simulink library "Vessel"  (R2023a)
settings: Solver=VariableStepAuto  StartTime=0.0  StopTime=10.0  RelTol=1e-3
undefined symbols (not defined in the file): A_ann_aor, alpha1, alpha2, atrium_ventricle, BSA, control, conversion_factor, DAP, DLVP, DP_close_aor, DP_open_aor, DPP, DRVP, E0, E_max, E_min, E_sa_0, E_sv_0, eta, g, K_vc_aor, K_vo_aor, l, L0, lambda, m1, m2, M_rg_aor, M_st_aor, MAP, MPP, n, P0, p_septum_on_off, p_th_on_off, phi, PVR, Q_max, rho, SAP, SI, sigma, SLVP, SPP, SRVP, SVR, t_delay, Ts, UVV_0, V0, V_0, V_max, V_tot, Y_aorta, Y_control
libraries: $bdroot x100, simulink x39, dspsigops x20, slpidlib x11, eeGeneralControl x2, dspstat3 x1
(part 2 of 4)

== system Vessel/DLVP control1 ==
  DLVP(t) : Inport
  Constant : Constant  Value=DLVP_0
  Constant1 : Constant  Value=onoff
  Data Store Write : DataStoreWrite  DataStoreName=K_LV_Emin  IndexOptions=Index vector (dialog)  Indices=1  OutputSizes=1
  IsZero : simulink/Logic and Bit Operations/Compare To Zero  relop=~=  OutDataTypeStr=boolean
      settings: LibrarySourceBlock=|
      | simulink/Quick Insert/Logic and Bit
      | Operations/IsZero
  IsZero2 : simulink/Logic and Bit Operations/Compare To Zero  relop===  OutDataTypeStr=boolean
      settings: LibrarySourceBlock=|
      | simulink/Quick Insert/Logic and Bit
      | Operations/IsZero
  OR : Logic  Operator=OR  IconShape=distinctive  AllPortsSameDT=off  OutDataTypeStr=boolean
  PID Controller : slpidlib/PID Controller  Controller=PI  Form=Parallel  TimeDomain=Discrete-time  UseExternalTs=off  SampleTime=dt  IntegratorMethod=Forward Euler  FilterMethod=Forward Euler  ControllerParametersSource=internal  P=0.005  I=0.005  UseKiTs=off  D=0.01  N=100  UseFilter=on  TunerSelectOption=Transfer Function Based (PID Tuner App)  InitialConditionSource=internal  InitialConditionForIntegrator=0  InitialConditionForFilter=0  DifferentiatorICPrevScaledInput=0  ExternalReset=either  TrackingMode=off  Kt=1  LimitOutput=on  SatLimitsSource=internal  UpperSaturationLimit=2  LowerSaturationLimit=-0.99  LinearizeAsGain=on  AntiWindupMode=none  Kb=1  LimitIntegrator=off  UpperIntegratorSaturationLimit=inf  LowerIntegratorSaturationLimit=-inf  POutMin=[]  POutMax=[]  IOutMin=[]  IOutMax=[]  DOutMin=[]  DOutMax=[]  NOutMin=[]  NOutMax=[]  SumOutMin=[]  SumOutMax=[]  SaturationOutMin=[]  SaturationOutMax=[]  PParamMin=[]  PParamMax=[]  IParamMin=[]  IParamMax=[]  DParamMin=[]  DParamMax=[]  NParamMin=[]  NParamMax=[]  KbParamMin=[]  KbParamMax=[]  KtParamMin=[]  KtParamMax=[]  KbOutMin=[]  KbOutMax=[]  KtOutMin=[]  KtOutMax=[]  IntegratorOutMin=[]  IntegratorOutMax=[]  FilterOutMin=[]  FilterOutMax=[]  SumI1OutMin=[]  SumI1OutMax=[]  SumI2OutMin=[]  SumI2OutMax=[]  SumI3OutMin=[]  SumI3OutMax=[]  SumI4OutMin=[]  SumI4OutMax=[]  SumDOutMin=[]  SumDOutMax=[]  DifferentiatorOutMin=[]  DifferentiatorOutMax=[]  FilterDiffOutCoefMin=[]  FilterDiffOutCoefMax=[]  ReciprocalOutMin=[]  ReciprocalOutMax=[]  SumDenOutMin=[]  SumDenOutMax=[]  SumNumOutMin=[]  SumNumOutMax=[]  DivideOutMin=[]  DivideOutMax=[]  UdiffTsProdOutMin=[]  UdiffTsProdOutMax=[]  NTsProdOutMin=[]  NTsProdOutMax=[]  UintegralTsProdOutMin=[]  UintegralTsProdOutMax=[]  UngainTsProdOutMin=[]  UngainTsProdOutMax=[]  ClampingZeroOutDataTypeStr=Inherit: Inherit via back propagation  ClampingZeroOutMin=[]  ClampingZeroOutMax=[]  FilterDenConstantOutDataTypeStr=Inherit: Inherit via back propagation  FilterDenConstantOutMin=[]  FilterDenConstantOutMax=[]  PCopyOutDataTypeStr=Inherit: Inherit via back propagation  PCopyOutMin=[]  PCopyOutMax=[]  NCopyOutDataTypeStr=Inherit: Inherit via back propagation  NCopyOutMin=[]  NCopyOutMax=[]  IntegratorContinuousStateAttributes=''  IntegratorStateMustResolveToSignalObject=off  IntegratorRTWStateStorageClass=Auto  FilterContinuousStateAttributes=''  FilterStateMustResolveToSignalObject=off  FilterRTWStateStorageClass=Auto  ParallelPVariant=InternalParameters  IdealPVariant=Disabled  IVariant=InternalParameters  DVariant=Disabled  IntegratorVariant=Discrete  SatVariant=Enabled  AWVariant=Passthrough  PCopyVariant=Disabled  TRVariant=Disabled  FdbkBlocksVariant=Forward  IdealPFdbkVariant=Disabled  SatFdbkVariant=Disabled  DerivativeFilterVariant=Disabled  NVariant=Disabled  NCopyVariant=Disabled_SignalSpec  FilterICVariant=Disabled  IntegratorICVariant=InternalICs  ExternalResetVariant=ExternalReset  TRSumVariant=Passthrough  SumFdbkVariant=Disabled  SumVariant=Sum_PI  TsampFilterVariant=InternalTs  TsampNgainVariant=Passthrough  TsampIntegralVariant=Disabled_SignalSpec  ExternalSaturationOutDataTypeStr=Inherit: Same as second input
  Product : Product
  Subsystem : $bdroot/SLVP control/Subsystem  SystemSampleTime=-1  SSRTWFcnClass=[]  VariantActivationTime=update diagram  Latency=0  AutoFrameSizeCalculation=off
      settings: LibrarySourceBlock=Vessel/SLVP control/Subsystem
  Subtract : Sum  Inputs=+-
  Switch : Switch  Criteria=u2 > Threshold  SaturateOnIntegerOverflow=off  InputSameDT=off
  Switch1 : Switch  Criteria=u2 > Threshold  SaturateOnIntegerOverflow=off  InputSameDT=off
  wires:
  Subtract/1 -> PID Controller/1  "V(t)"
  Constant/1 -> Switch1/3
  [DLVP] -> IsZero2/1, Switch/3
  Switch/1 -> Subtract/2
  IsZero2/1 -> Switch/2
  DLVP(t)/1 -> Switch1/2, IsZero/1, Switch1/1
  Switch1/1 -> Subtract/1, Switch/1
  Product/1 -> Subsystem/2
  IsZero/1 -> OR/2
  Constant1/1 -> OR/1
  OR/1 -> Subsystem/1, Product/1, PID Controller/2
  PID Controller/1 -> Product/2
  Subsystem/1 -> Data Store Write/1

== system Vessel/DRVP control ==
  DRVP(t) : Inport
  Constant : Constant  Value=DRVP_0
  Constant1 : Constant  Value=onoff
  Data Store Write : DataStoreWrite  DataStoreName=K_RV_Emin  IndexOptions=Index vector (dialog)  Indices=1  OutputSizes=1
  IsZero : simulink/Logic and Bit Operations/Compare To Zero  relop=~=  OutDataTypeStr=boolean
      settings: LibrarySourceBlock=|
      | simulink/Quick Insert/Logic and Bit
      | Operations/IsZero
  IsZero2 : simulink/Logic and Bit Operations/Compare To Zero  relop===  OutDataTypeStr=boolean
      settings: LibrarySourceBlock=|
      | simulink/Quick Insert/Logic and Bit
      | Operations/IsZero
  OR : Logic  Operator=OR  IconShape=distinctive  AllPortsSameDT=off  OutDataTypeStr=boolean
  PID Controller : slpidlib/PID Controller  Controller=PI  Form=Parallel  TimeDomain=Discrete-time  UseExternalTs=off  SampleTime=dt  IntegratorMethod=Forward Euler  FilterMethod=Forward Euler  ControllerParametersSource=internal  P=0.005  I=0.005  UseKiTs=off  D=0.01  N=100  UseFilter=on  TunerSelectOption=Transfer Function Based (PID Tuner App)  InitialConditionSource=internal  InitialConditionForIntegrator=0  InitialConditionForFilter=0  DifferentiatorICPrevScaledInput=0  ExternalReset=either  TrackingMode=off  Kt=1  LimitOutput=on  SatLimitsSource=internal  UpperSaturationLimit=2  LowerSaturationLimit=-0.99  LinearizeAsGain=on  AntiWindupMode=none  Kb=1  LimitIntegrator=off  UpperIntegratorSaturationLimit=inf  LowerIntegratorSaturationLimit=-inf  POutMin=[]  POutMax=[]  IOutMin=[]  IOutMax=[]  DOutMin=[]  DOutMax=[]  NOutMin=[]  NOutMax=[]  SumOutMin=[]  SumOutMax=[]  SaturationOutMin=[]  SaturationOutMax=[]  PParamMin=[]  PParamMax=[]  IParamMin=[]  IParamMax=[]  DParamMin=[]  DParamMax=[]  NParamMin=[]  NParamMax=[]  KbParamMin=[]  KbParamMax=[]  KtParamMin=[]  KtParamMax=[]  KbOutMin=[]  KbOutMax=[]  KtOutMin=[]  KtOutMax=[]  IntegratorOutMin=[]  IntegratorOutMax=[]  FilterOutMin=[]  FilterOutMax=[]  SumI1OutMin=[]  SumI1OutMax=[]  SumI2OutMin=[]  SumI2OutMax=[]  SumI3OutMin=[]  SumI3OutMax=[]  SumI4OutMin=[]  SumI4OutMax=[]  SumDOutMin=[]  SumDOutMax=[]  DifferentiatorOutMin=[]  DifferentiatorOutMax=[]  FilterDiffOutCoefMin=[]  FilterDiffOutCoefMax=[]  ReciprocalOutMin=[]  ReciprocalOutMax=[]  SumDenOutMin=[]  SumDenOutMax=[]  SumNumOutMin=[]  SumNumOutMax=[]  DivideOutMin=[]  DivideOutMax=[]  UdiffTsProdOutMin=[]  UdiffTsProdOutMax=[]  NTsProdOutMin=[]  NTsProdOutMax=[]  UintegralTsProdOutMin=[]  UintegralTsProdOutMax=[]  UngainTsProdOutMin=[]  UngainTsProdOutMax=[]  ClampingZeroOutDataTypeStr=Inherit: Inherit via back propagation  ClampingZeroOutMin=[]  ClampingZeroOutMax=[]  FilterDenConstantOutDataTypeStr=Inherit: Inherit via back propagation  FilterDenConstantOutMin=[]  FilterDenConstantOutMax=[]  PCopyOutDataTypeStr=Inherit: Inherit via back propagation  PCopyOutMin=[]  PCopyOutMax=[]  NCopyOutDataTypeStr=Inherit: Inherit via back propagation  NCopyOutMin=[]  NCopyOutMax=[]  IntegratorContinuousStateAttributes=''  IntegratorStateMustResolveToSignalObject=off  IntegratorRTWStateStorageClass=Auto  FilterContinuousStateAttributes=''  FilterStateMustResolveToSignalObject=off  FilterRTWStateStorageClass=Auto  ParallelPVariant=InternalParameters  IdealPVariant=Disabled  IVariant=InternalParameters  DVariant=Disabled  IntegratorVariant=Discrete  SatVariant=Enabled  AWVariant=Passthrough  PCopyVariant=Disabled  TRVariant=Disabled  FdbkBlocksVariant=Forward  IdealPFdbkVariant=Disabled  SatFdbkVariant=Disabled  DerivativeFilterVariant=Disabled  NVariant=Disabled  NCopyVariant=Disabled_SignalSpec  FilterICVariant=Disabled  IntegratorICVariant=InternalICs  ExternalResetVariant=ExternalReset  TRSumVariant=Passthrough  SumFdbkVariant=Disabled  SumVariant=Sum_PI  TsampFilterVariant=InternalTs  TsampNgainVariant=Passthrough  TsampIntegralVariant=Disabled_SignalSpec  ExternalSaturationOutDataTypeStr=Inherit: Same as second input
  Product : Product
  Subsystem : $bdroot/SLVP control/Subsystem  SystemSampleTime=-1  VariantActivationTime=update diagram  Latency=0  AutoFrameSizeCalculation=off
  Subtract : Sum  Inputs=+-
  Switch : Switch  Criteria=u2 > Threshold  SaturateOnIntegerOverflow=off  InputSameDT=off
  Switch1 : Switch  Criteria=u2 > Threshold  SaturateOnIntegerOverflow=off  InputSameDT=off
  wires:
  PID Controller/1 -> Product/2
  OR/1 -> Subsystem/1, PID Controller/2, Product/1
  Constant1/1 -> OR/1
  IsZero/1 -> OR/2
  Product/1 -> Subsystem/2
  Switch1/1 -> Switch/1, Subtract/1
  DRVP(t)/1 -> Switch1/1, IsZero/1, Switch1/2
  IsZero2/1 -> Switch/2
  Switch/1 -> Subtract/2
  [DRVP] -> IsZero2/1, Switch/3
  Constant/1 -> Switch1/3
  Subtract/1 -> PID Controller/1  "V(t)"
  Subsystem/1 -> Data Store Write/1

== system Vessel/Delta to Star conversion ==
  R1 : Inport
  R2 : Inport  Port=2
  R3 : Inport  Port=3
  Add : Sum  Inputs=3
  Divide : Product  Inputs=*/
  Divide1 : Product  Inputs=*/
  Divide2 : Product  Inputs=*/
  Product : Product
  Product1 : Product
  Product2 : Product
  Ra : Outport
  Rb : Outport  Port=2
  Rc : Outport  Port=3
  wires:
  Product1/1 -> Divide/1
  Product2/1 -> Divide1/1
  R1/1 -> Add/2, Product2/1, Product/1
  R2/1 -> Add/3, Product/2, Product1/1
  R3/1 -> Product1/2, Add/1, Product2/2
  Divide/1 -> Ra/1
  Divide1/1 -> Rb/1
  Divide2/1 -> Rc/1
  Add/1 -> Divide1/2, Divide/2, Divide2/2
  Product/1 -> Divide2/1

== system Vessel/Diastolic Pressur ==
  P_in : Inport
  MinMax Running Resettable : simulink/Math Operations/MinMax Running Resettable  Function=min  vinit=300
      settings: AttributesFormatString=%<vinit>
  Pulse Generator1 : DiscretePulseGenerator  PulseType=Time based  TimeSource=Use external signal  Period=100  PulseWidth=1e-3
  Sample and Hold1 : dspsigops/Sample and Hold  trig=Rising edge  initCond=0  latchinput=on
  P_dys : Outport
  wires:
  MinMax Running Resettable/1 -> Sample and Hold1/1
  [t_b] -> Pulse Generator1/1
  P_in/1 -> MinMax Running Resettable/1
  Pulse Generator1/1 -> MinMax Running Resettable/2, Sample and Hold1/Trigger
  Sample and Hold1/1 -> P_dys/1

== system Vessel/Gain ==
  Add : Sum
  Constant : Constant
  Constant1 : Constant  Commented=on  Value=0
  Constant2 : Constant  Commented=on  Value=0
  Constant6 : Constant  Commented=on  Value=control
  Data Store Read : DataStoreRead  Commented=on  DataStoreName=K_svr  IndexOptions=Index vector (dialog)  Indices=1  OutputSizes=1
  Data Store Read1 : DataStoreRead  Commented=on  DataStoreName=K_pvr  IndexOptions=Index vector (dialog)  Indices=1  OutputSizes=1
  Data Store Read2 : DataStoreRead  Commented=on  DataStoreName=K_uvv  IndexOptions=Index vector (dialog)  Indices=1  OutputSizes=1
  Multiport Switch : MultiPortSwitch  Commented=on  Inputs=5  SaturateOnIntegerOverflow=off  InputSameDT=off
  Gain : Outport
  wires:
  Constant2/1 -> Multiport Switch/5
  Constant6/1 -> Multiport Switch/1
  Data Store Read/1 -> Multiport Switch/2
  Add/1 -> Gain/1
  Data Store Read1/1 -> Multiport Switch/3
  Data Store Read2/1 -> Multiport Switch/4
  Constant1/1 -> Multiport Switch/6
  Constant/1 -> Add/1
  Multiport Switch/1 -> Add/2

== system Vessel/Gain UVV ==
  V0 : Inport
  Add : Sum
  Constant : Constant
  Constant1 : Constant  Commented=on  Value=3
  Constant2 : Constant  Commented=on  Value=0
  Constant3 : Constant  Value=0
  Constant4 : Constant  Value=0
  Constant5 : Constant  Value=control
  Constant6 : Constant  Commented=on  Value=control
  Data Store Read : DataStoreRead  DataStoreName=K_svr  IndexOptions=Index vector (dialog)  Indices=1  OutputSizes=1
  Data Store Read1 : DataStoreRead  DataStoreName=K_pvr  IndexOptions=Index vector (dialog)  Indices=1  OutputSizes=1
  Data Store Read2 : DataStoreRead  Commented=on  DataStoreName=K_uvv  IndexOptions=Index vector (dialog)  Indices=1  OutputSizes=1
  Data Store Read3 : DataStoreRead  DataStoreName=K_uvv  IndexOptions=Index vector (dialog)  Indices=1  OutputSizes=1
  Equal : RelationalOperator  Commented=on  Operator===  OutDataTypeStr=boolean  RndMeth=Simplest  InputSameDT=off
  Multiport Switch : MultiPortSwitch  Inputs=5  SaturateOnIntegerOverflow=off  InputSameDT=off
  Product : Product
  Switch : Switch  Commented=on  Criteria=u2 ~= 0  Threshold=3  SaturateOnIntegerOverflow=off  InputSameDT=off
  V0* : Outport
  wires:
  Multiport Switch/1 -> Add/2
  Constant/1 -> Add/1
  Add/1 -> Product/2
  Constant6/1 -> Equal/1
  Constant1/1 -> Equal/2
  Equal/1 -> Switch/2
  Data Store Read2/1 -> Switch/1
  V0/1 -> Product/1
  Product/1 -> V0*/1
  Constant2/1 -> Switch/3
  Constant5/1 -> Multiport Switch/1
  Data Store Read1/1 -> Multiport Switch/3
  Constant4/1 -> Multiport Switch/5
  Data Store Read3/1 -> Multiport Switch/4
  Data Store Read/1 -> Multiport Switch/2
  Constant3/1 -> Multiport Switch/6

== system Vessel/Gain_E_max ==
  E_max : Inport
  Add : Sum
  Constant : Constant
  Constant1 : Constant  Value=0
  Constant2 : Constant  Value=0
  Constant6 : Constant  Value=control
  Data Store Read : DataStoreRead  DataStoreName=K_RA_Emax  IndexOptions=Index vector (dialog)  Indices=1  OutputSizes=1
  Data Store Read1 : DataStoreRead  DataStoreName=K_RV_Emax  IndexOptions=Index vector (dialog)  Indices=1  OutputSizes=1
  Data Store Read2 : DataStoreRead  DataStoreName=K_LA_Emax  IndexOptions=Index vector (dialog)  Indices=1  OutputSizes=1
  Data Store Read3 : DataStoreRead  DataStoreName=K_LV_Emax  IndexOptions=Index vector (dialog)  Indices=1  OutputSizes=1
  Multiport Switch : MultiPortSwitch  Inputs=6  SaturateOnIntegerOverflow=off  InputSameDT=off
  Product : Product
  E_max* : Outport
  wires:
  Multiport Switch/1 -> Add/2
  Constant/1 -> Add/1
  Constant1/1 -> Multiport Switch/7
  Data Store Read2/1 -> Multiport Switch/4
  Data Store Read1/1 -> Multiport Switch/3
  Add/1 -> Product/2
  Data Store Read/1 -> Multiport Switch/2
  Constant6/1 -> Multiport Switch/1
  Data Store Read3/1 -> Multiport Switch/5
  Constant2/1 -> Multiport Switch/6
  Product/1 -> E_max*/1
  E_max/1 -> Product/1

== system Vessel/Gain_E_min ==
  E_min : Inport
  Add : Sum
  Constant : Constant
  Constant1 : Constant  Value=0
  Constant2 : Constant  Value=0
  Constant6 : Constant  Value=control
  Data Store Read : DataStoreRead  DataStoreName=K_RA_Emin  IndexOptions=Index vector (dialog)  Indices=1  OutputSizes=1
  Data Store Read1 : DataStoreRead  DataStoreName=K_RV_Emin  IndexOptions=Index vector (dialog)  Indices=1  OutputSizes=1
  Data Store Read2 : DataStoreRead  DataStoreName=K_LA_Emin  IndexOptions=Index vector (dialog)  Indices=1  OutputSizes=1
  Data Store Read3 : DataStoreRead  DataStoreName=K_LV_Emin  IndexOptions=Index vector (dialog)  Indices=1  OutputSizes=1
  Multiport Switch : MultiPortSwitch  Inputs=6  SaturateOnIntegerOverflow=off  InputSameDT=off
  Product : Product
  E_min* : Outport
  wires:
  E_min/1 -> Product/1
  Product/1 -> E_min*/1
  Constant2/1 -> Multiport Switch/6
  Data Store Read3/1 -> Multiport Switch/5
  Constant6/1 -> Multiport Switch/1
  Data Store Read/1 -> Multiport Switch/2
  Add/1 -> Product/2
  Data Store Read1/1 -> Multiport Switch/3
  Data Store Read2/1 -> Multiport Switch/4
  Constant1/1 -> Multiport Switch/7
  Constant/1 -> Add/1
  Multiport Switch/1 -> Add/2

== system Vessel/Gain_Y ==
  Y : Inport
  Add : Sum
  Constant : Constant
  Constant1 : Constant  Value=0
  Constant2 : Constant  Value=0
  Constant6 : Constant  Value=Y_control
  Data Store Read : DataStoreRead  DataStoreName=K_Y_aorta  IndexOptions=Index vector (dialog)  Indices=1  OutputSizes=1
  Data Store Read1 : DataStoreRead  DataStoreName=K_Y_systemic_veins  IndexOptions=Index vector (dialog)  Indices=1  OutputSizes=1
  Data Store Read2 : DataStoreRead  DataStoreName=K_Y_pulmonary_arteries  IndexOptions=Index vector (dialog)  Indices=1  OutputSizes=1
  Data Store Read3 : DataStoreRead  DataStoreName=K_Y_pulmonary_veins  IndexOptions=Index vector (dialog)  Indices=1  OutputSizes=1
  Multiport Switch : MultiPortSwitch  Inputs=6  SaturateOnIntegerOverflow=off  InputSameDT=off
  Product : Product
  Y* : Outport
  wires:
  Y/1 -> Product/1
  Product/1 -> Y*/1
  Constant2/1 -> Multiport Switch/6
  Data Store Read3/1 -> Multiport Switch/5
  Constant6/1 -> Multiport Switch/1
  Data Store Read/1 -> Multiport Switch/2
  Add/1 -> Product/2
  Data Store Read1/1 -> Multiport Switch/3
  Data Store Read2/1 -> Multiport Switch/4
  Constant1/1 -> Multiport Switch/7
  Constant/1 -> Add/1
  Multiport Switch/1 -> Add/2

== system Vessel/Heart Chamber1 ==
  Q_Input : Inport
  Q_Output : Inport  Port=2
  P_other : Inport  Port=3
  Constant : Constant  Value=p_septum_on_off
  Constant10 : Constant  Value=R_wall
  Constant11 : Constant  Value=v_o
  Constant13 : Constant  Value=V_0
  Delay : Delay  DelayLength=1
  Delay1 : Delay  DelayLength=1  InitialCondition=0
  Integrator : Integrator  InitialConditionSource=external  LimitOutput=on  UpperSaturationLimit=V_max  LowerSaturationLimit=0
  Pericardial pressure : Subsystem
  Product1 : Product  Inputs=3
  Product2 : Product
  Sum1 : Sum  Inputs=+-
  Sum2 : Sum  Inputs=+++
  Sum3 : Sum  Inputs=+-
  Switch : Switch  Criteria=u2 > Threshold  SaturateOnIntegerOverflow=off  InputSameDT=off
  Time varying elastance1 : $bdroot/Time varying elastance1  SystemSampleTime=-1  VariantActivationTime=update diagram  Latency=0  AutoFrameSizeCalculation=off
  Transeptal pressure : $bdroot/Transeptal pressure  SystemSampleTime=-1  VariantActivationTime=update diagram  Latency=0  AutoFrameSizeCalculation=off
  V_ed_new : $bdroot/V_ed_new  SystemSampleTime=-1  VariantActivationTime=update diagram  Latency=0  AutoFrameSizeCalculation=off
  P_Output : Outport
  V : Outport  Port=2
  wires:
  Product2/1 -> Switch/3
  Sum3/1 -> Transeptal pressure/1, Product2/1  "V-V_0"
  Constant13/1 -> Sum3/2
  Integrator/1 -> V_ed_new/1, Time varying elastance1/2, V/1, Sum3/1  "V"
  Constant11/1 -> Integrator/2
  Constant10/1 -> Product1/3
  Sum2/1 -> Delay1/1  "P_chamber"
  Q_Input/1 -> Sum1/1
  Sum1/1 -> Delay/1, Integrator/1  "V'"
  Pericardial pressure/1(P_pc) -> Sum2/3  "P_pc"
  V_ed_new/1 -> Time varying elastance1/1
  Transeptal pressure/1 -> Switch/1
  Constant/1 -> Switch/2
  Switch/1 -> Product1/1, Sum2/1
  P_other/1 -> Transeptal pressure/3
  Delay/1 -> Product1/2
  [V_pc] -> Pericardial pressure/1(Vpc)
  Time varying elastance1/1 -> Product2/2, Transeptal pressure/2
  Product1/1 -> Sum2/2
  Q_Output/1 -> Sum1/2, Time varying elastance1/3
  Delay1/1 -> P_Output/1

== system Vessel/Inductance ==
  r(t) : Inport
  Gain1 : Gain  Gain=rho*l/pi/n/g/conversion_factor
  Math Function : Math  Operator=reciprocal
  Power1 : Math  Operator=square
  L(t) : Outport
  wires:
  Math Function/1 -> Gain1/1
  r(t)/1 -> Power1/1
  Power1/1 -> Math Function/1
  Gain1/1 -> L(t)/1  "L(t)"

== system Vessel/Intrathoracic Pressure ==
  Add : Sum  Inputs=-+
  Add1 : Sum
  Breathing cycle : Subsystem
  Constant : Constant  Value=t_exp
  Constant1 : Constant
  Constant2 : Constant  Value=p_itb
  Constant4 : Constant  Value=t_exp
  Exp : Math
  Exp1 : Math
  Subtract : Sum  Inputs=+-
  Subtract1 : Sum  Inputs=+-
  Switch : Switch  SaturateOnIntegerOverflow=off  InputSameDT=off
  To Workspace4 : ToWorkspace  VariableName=P_Ao1  SampleTime=-1
  amplitude : Gain  Gain=p_ita
  amplitude1 : Gain  Gain=p_ita
  expiration : Gain  Gain=-1/tau_exp
  inspiration : Gain  Gain=-1/tau_insp
  P_ith : Outport
  tag scope: P_ith=global
  wires:
  Switch/1 -> Add1/1
  amplitude1/1 -> Switch/3
  Constant2/1 -> Add1/2
  Add/1 -> amplitude1/1
  Exp/1 -> amplitude/1
  Constant/1 -> Subtract/2
  Subtract/1 -> Switch/2
  Exp1/1 -> Add/1
  expiration/1 -> Exp1/1
  inspiration/1 -> Exp/1
  [t_breathing] -> Subtract/1
  Constant1/1 -> Add/2
  Subtract1/1 -> inspiration/1
  Constant4/1 -> Subtract1/2
  amplitude/1 -> Switch/1
  [t_breathing] -> expiration/1
  [t_breathing] -> Subtract1/1
  Add1/1 -> To Workspace4/1, [P_ith], P_ith/1

== system Vessel/MAP ==
  P_ao : Inport
  Data Store Read1 : DataStoreRead  DataStoreName=T  IndexOptions=Index vector (dialog)  Indices=1  OutputSizes=1
  Divide : Product  Inputs=/*
  Integrator : Integrator  ExternalReset=falling
  Pulse Generator : DiscretePulseGenerator  PulseType=Time based  TimeSource=Use external signal  Period=100  PulseWidth=1e-3
  Sample and Hold : dspsigops/Sample and Hold  trig=Rising edge  initCond=0  latchinput=off
  MAP : Outport
  wires:
  P_ao/1 -> Integrator/1
  Data Store Read1/1 -> Divide/1
  Divide/1 -> MAP/1
  [t_b] -> Pulse Generator/1
  Pulse Generator/1 -> Sample and Hold/Trigger, Integrator/2
  Integrator/1 -> Sample and Hold/1
  Sample and Hold/1 -> Divide/2

== system Vessel/MAP control ==
  MAP(t) : Inport
  Constant : Constant  Value=MAP_0
  Constant1 : Constant  Value=onoff
  Data Store Write : DataStoreWrite  DataStoreName=K_LV_Emax  IndexOptions=Index vector (dialog)  Indices=1  OutputSizes=1
  IsZero : simulink/Logic and Bit Operations/Compare To Zero  relop=~=  OutDataTypeStr=boolean
      settings: LibrarySourceBlock=|
      | simulink/Quick Insert/Logic and Bit
      | Operations/IsZero
  IsZero2 : simulink/Logic and Bit Operations/Compare To Zero  relop===  OutDataTypeStr=boolean
      settings: LibrarySourceBlock=|
      | simulink/Quick Insert/Logic and Bit
      | Operations/IsZero
  OR : Logic  Operator=OR  IconShape=distinctive  AllPortsSameDT=off  OutDataTypeStr=boolean
  PID Controller : slpidlib/PID Controller  Controller=PI  Form=Parallel  TimeDomain=Discrete-time  UseExternalTs=off  SampleTime=dt  IntegratorMethod=Forward Euler  FilterMethod=Forward Euler  ControllerParametersSource=internal  P=0.01  I=0.01  UseKiTs=off  D=0.01  N=100  UseFilter=on  TunerSelectOption=Transfer Function Based (PID Tuner App)  InitialConditionSource=internal  InitialConditionForIntegrator=0  InitialConditionForFilter=0  DifferentiatorICPrevScaledInput=0  ExternalReset=either  TrackingMode=off  Kt=1  LimitOutput=on  SatLimitsSource=internal  UpperSaturationLimit=2  LowerSaturationLimit=-0.99  LinearizeAsGain=on  AntiWindupMode=none  Kb=1  LimitIntegrator=off  UpperIntegratorSaturationLimit=inf  LowerIntegratorSaturationLimit=-inf  POutMin=[]  POutMax=[]  IOutMin=[]  IOutMax=[]  DOutMin=[]  DOutMax=[]  NOutMin=[]  NOutMax=[]  SumOutMin=[]  SumOutMax=[]  SaturationOutMin=[]  SaturationOutMax=[]  PParamMin=[]  PParamMax=[]  IParamMin=[]  IParamMax=[]  DParamMin=[]  DParamMax=[]  NParamMin=[]  NParamMax=[]  KbParamMin=[]  KbParamMax=[]  KtParamMin=[]  KtParamMax=[]  KbOutMin=[]  KbOutMax=[]  KtOutMin=[]  KtOutMax=[]  IntegratorOutMin=[]  IntegratorOutMax=[]  FilterOutMin=[]  FilterOutMax=[]  SumI1OutMin=[]  SumI1OutMax=[]  SumI2OutMin=[]  SumI2OutMax=[]  SumI3OutMin=[]  SumI3OutMax=[]  SumI4OutMin=[]  SumI4OutMax=[]  SumDOutMin=[]  SumDOutMax=[]  DifferentiatorOutMin=[]  DifferentiatorOutMax=[]  FilterDiffOutCoefMin=[]  FilterDiffOutCoefMax=[]  ReciprocalOutMin=[]  ReciprocalOutMax=[]  SumDenOutMin=[]  SumDenOutMax=[]  SumNumOutMin=[]  SumNumOutMax=[]  DivideOutMin=[]  DivideOutMax=[]  UdiffTsProdOutMin=[]  UdiffTsProdOutMax=[]  NTsProdOutMin=[]  NTsProdOutMax=[]  UintegralTsProdOutMin=[]  UintegralTsProdOutMax=[]  UngainTsProdOutMin=[]  UngainTsProdOutMax=[]  ClampingZeroOutDataTypeStr=Inherit: Inherit via back propagation  ClampingZeroOutMin=[]  ClampingZeroOutMax=[]  FilterDenConstantOutDataTypeStr=Inherit: Inherit via back propagation  FilterDenConstantOutMin=[]  FilterDenConstantOutMax=[]  PCopyOutDataTypeStr=Inherit: Inherit via back propagation  PCopyOutMin=[]  PCopyOutMax=[]  NCopyOutDataTypeStr=Inherit: Inherit via back propagation  NCopyOutMin=[]  NCopyOutMax=[]  IntegratorContinuousStateAttributes=''  IntegratorStateMustResolveToSignalObject=off  IntegratorRTWStateStorageClass=Auto  FilterContinuousStateAttributes=''  FilterStateMustResolveToSignalObject=off  FilterRTWStateStorageClass=Auto  ParallelPVariant=InternalParameters  IdealPVariant=Disabled  IVariant=InternalParameters  DVariant=Disabled  IntegratorVariant=Discrete  SatVariant=Enabled  AWVariant=Passthrough  PCopyVariant=Disabled  TRVariant=Disabled  FdbkBlocksVariant=Forward  IdealPFdbkVariant=Disabled  SatFdbkVariant=Disabled  DerivativeFilterVariant=Disabled  NVariant=Disabled  NCopyVariant=Disabled_SignalSpec  FilterICVariant=Disabled  IntegratorICVariant=InternalICs  ExternalResetVariant=ExternalReset  TRSumVariant=Passthrough  SumFdbkVariant=Disabled  SumVariant=Sum_PI  TsampFilterVariant=InternalTs  TsampNgainVariant=Passthrough  TsampIntegralVariant=Disabled_SignalSpec  ExternalSaturationOutDataTypeStr=Inherit: Same as second input
  Product : Product
  Subsystem : $bdroot/SLVP control/Subsystem  SystemSampleTime=-1  VariantActivationTime=update diagram  Latency=0  AutoFrameSizeCalculation=off
  Subtract : Sum  Inputs=+-
  Switch : Switch  Criteria=u2 > Threshold  SaturateOnIntegerOverflow=off  InputSameDT=off
  Switch1 : Switch  Criteria=u2 > Threshold  SaturateOnIntegerOverflow=off  InputSameDT=off
  wires:
  Subtract/1 -> PID Controller/1  "V(t)"
  Constant/1 -> Switch1/3
  [MAP] -> IsZero2/1, Switch/3
  Switch/1 -> Subtract/2
  IsZero2/1 -> Switch/2
  MAP(t)/1 -> Switch1/2, IsZero/1, Switch1/1
  Switch1/1 -> Subtract/1, Switch/1
  Product/1 -> Subsystem/2
  IsZero/1 -> OR/2
  Constant1/1 -> OR/1
  OR/1 -> Subsystem/1, Product/1, PID Controller/2
  PID Controller/1 -> Product/2
  Subsystem/1 -> Data Store Write/1

== system Vessel/MPP control ==
  MPP(t) : Inport
  Constant : Constant  Value=MPP_0
  Constant1 : Constant  Value=onoff
  Data Store Write : DataStoreWrite  DataStoreName=K_RV_Emax  IndexOptions=Index vector (dialog)  Indices=1  OutputSizes=1
  IsZero : simulink/Logic and Bit Operations/Compare To Zero  relop=~=  OutDataTypeStr=boolean
      settings: LibrarySourceBlock=|
      | simulink/Quick Insert/Logic and Bit
      | Operations/IsZero
  IsZero2 : simulink/Logic and Bit Operations/Compare To Zero  relop===  OutDataTypeStr=boolean
      settings: LibrarySourceBlock=|
      | simulink/Quick Insert/Logic and Bit
      | Operations/IsZero
  OR : Logic  Operator=OR  IconShape=distinctive  AllPortsSameDT=off  OutDataTypeStr=boolean
  PID Controller : slpidlib/PID Controller  Controller=PI  Form=Parallel  TimeDomain=Discrete-time  UseExternalTs=off  SampleTime=dt  IntegratorMethod=Forward Euler  FilterMethod=Forward Euler  ControllerParametersSource=internal  P=0.005  I=0.005  UseKiTs=off  D=0.01  N=100  UseFilter=on  TunerSelectOption=Transfer Function Based (PID Tuner App)  InitialConditionSource=internal  InitialConditionForIntegrator=0  InitialConditionForFilter=0  DifferentiatorICPrevScaledInput=0  ExternalReset=either  TrackingMode=off  Kt=1  LimitOutput=on  SatLimitsSource=internal  UpperSaturationLimit=2  LowerSaturationLimit=-0.99  LinearizeAsGain=on  AntiWindupMode=none  Kb=1  LimitIntegrator=off  UpperIntegratorSaturationLimit=inf  LowerIntegratorSaturationLimit=-inf  POutMin=[]  POutMax=[]  IOutMin=[]  IOutMax=[]  DOutMin=[]  DOutMax=[]  NOutMin=[]  NOutMax=[]  SumOutMin=[]  SumOutMax=[]  SaturationOutMin=[]  SaturationOutMax=[]  PParamMin=[]  PParamMax=[]  IParamMin=[]  IParamMax=[]  DParamMin=[]  DParamMax=[]  NParamMin=[]  NParamMax=[]  KbParamMin=[]  KbParamMax=[]  KtParamMin=[]  KtParamMax=[]  KbOutMin=[]  KbOutMax=[]  KtOutMin=[]  KtOutMax=[]  IntegratorOutMin=[]  IntegratorOutMax=[]  FilterOutMin=[]  FilterOutMax=[]  SumI1OutMin=[]  SumI1OutMax=[]  SumI2OutMin=[]  SumI2OutMax=[]  SumI3OutMin=[]  SumI3OutMax=[]  SumI4OutMin=[]  SumI4OutMax=[]  SumDOutMin=[]  SumDOutMax=[]  DifferentiatorOutMin=[]  DifferentiatorOutMax=[]  FilterDiffOutCoefMin=[]  FilterDiffOutCoefMax=[]  ReciprocalOutMin=[]  ReciprocalOutMax=[]  SumDenOutMin=[]  SumDenOutMax=[]  SumNumOutMin=[]  SumNumOutMax=[]  DivideOutMin=[]  DivideOutMax=[]  UdiffTsProdOutMin=[]  UdiffTsProdOutMax=[]  NTsProdOutMin=[]  NTsProdOutMax=[]  UintegralTsProdOutMin=[]  UintegralTsProdOutMax=[]  UngainTsProdOutMin=[]  UngainTsProdOutMax=[]  ClampingZeroOutDataTypeStr=Inherit: Inherit via back propagation  ClampingZeroOutMin=[]  ClampingZeroOutMax=[]  FilterDenConstantOutDataTypeStr=Inherit: Inherit via back propagation  FilterDenConstantOutMin=[]  FilterDenConstantOutMax=[]  PCopyOutDataTypeStr=Inherit: Inherit via back propagation  PCopyOutMin=[]  PCopyOutMax=[]  NCopyOutDataTypeStr=Inherit: Inherit via back propagation  NCopyOutMin=[]  NCopyOutMax=[]  IntegratorContinuousStateAttributes=''  IntegratorStateMustResolveToSignalObject=off  IntegratorRTWStateStorageClass=Auto  FilterContinuousStateAttributes=''  FilterStateMustResolveToSignalObject=off  FilterRTWStateStorageClass=Auto  ParallelPVariant=InternalParameters  IdealPVariant=Disabled  IVariant=InternalParameters  DVariant=Disabled  IntegratorVariant=Discrete  SatVariant=Enabled  AWVariant=Passthrough  PCopyVariant=Disabled  TRVariant=Disabled  FdbkBlocksVariant=Forward  IdealPFdbkVariant=Disabled  SatFdbkVariant=Disabled  DerivativeFilterVariant=Disabled  NVariant=Disabled  NCopyVariant=Disabled_SignalSpec  FilterICVariant=Disabled  IntegratorICVariant=InternalICs  ExternalResetVariant=ExternalReset  TRSumVariant=Passthrough  SumFdbkVariant=Disabled  SumVariant=Sum_PI  TsampFilterVariant=InternalTs  TsampNgainVariant=Passthrough  TsampIntegralVariant=Disabled_SignalSpec  ExternalSaturationOutDataTypeStr=Inherit: Same as second input
  Product : Product
  Subsystem : $bdroot/SLVP control/Subsystem  SystemSampleTime=-1  VariantActivationTime=update diagram  Latency=0  AutoFrameSizeCalculation=off
  Subtract : Sum  Inputs=+-
  Switch : Switch  Criteria=u2 > Threshold  SaturateOnIntegerOverflow=off  InputSameDT=off
  Switch1 : Switch  Criteria=u2 > Threshold  SaturateOnIntegerOverflow=off  InputSameDT=off
  wires:
  PID Controller/1 -> Product/2
  OR/1 -> Subsystem/1, PID Controller/2, Product/1
  Constant1/1 -> OR/1
  IsZero/1 -> OR/2
  Product/1 -> Subsystem/2
  Switch1/1 -> Switch/1, Subtract/1
  MPP(t)/1 -> Switch1/1, IsZero/1, Switch1/2
  IsZero2/1 -> Switch/2
  Switch/1 -> Subtract/2
  [MPP] -> IsZero2/1, Switch/3
  Constant/1 -> Switch1/3
  Subtract/1 -> PID Controller/1  "V(t)"
  Subsystem/1 -> Data Store Write/1

== system Vessel/Omega ==
  V-V0 : Inport  Unit=mL
  L(t) : Inport  Port=2  Unit=mmHg*s^2/mL
  Constant : Constant  Value=E0
  Constant1 : Constant  Value=L0
  Constant9 : Constant  Value=lambda
  Product : Product
  Product9 : Product
  Sqrt : Sqrt
  Subsystem : Subsystem
  Switch1 : Switch  Criteria=u2 ~= 0  SaturateOnIntegerOverflow=off  InputSameDT=off
  Switch2 : Switch  Criteria=u2 > Threshold  SaturateOnIntegerOverflow=off  InputSameDT=off
  Ω : Outport
  wires:
  Product/1 -> Ω/1
  Constant9/1 -> Product/2
  V-V0/1 -> Switch1/2, Subsystem/1(V-V0)
  L(t)/1 -> Switch2/2, Switch2/1
  Switch1/1 -> Product9/1  "E(t)"
  Sqrt/1 -> Product/1
  Product9/1 -> Sqrt/1
  Subsystem/1(E(t)) -> Switch1/1  "E(t)"
  Constant/1 -> Switch1/3
  Switch2/1 -> Product9/2  "L(t)"
  Constant1/1 -> Switch2/3

== system Vessel/PVR Control ==
  PVR(t) : Inport
  Constant : Constant  Value=PVR_0
  Constant1 : Constant  Value=0
  Data Store Write : DataStoreWrite  DataStoreName=K_pvr  IndexOptions=Index vector (dialog)  Indices=1  OutputSizes=1
  IsZero1 : simulink/Logic and Bit Operations/Compare To Zero  relop=~=  OutDataTypeStr=boolean
      settings: LibrarySourceBlock=|
      | simulink/Quick Insert/Logic and Bit
      | Operations/IsZero
  K_pvr : Constant  Value=0
  MATLAB Function : MATLAB Function  TreatAsAtomicUnit=on
  OR : Logic  Operator=OR  IconShape=distinctive  AllPortsSameDT=off  OutDataTypeStr=boolean
  PID Controller : slpidlib/PID Controller  Controller=PI  Form=Parallel  TimeDomain=Continuous-time  UseExternalTs=off  SampleTime=-1  IntegratorMethod=Forward Euler  FilterMethod=Forward Euler  ControllerParametersSource=internal  P=0.3  I=0.3  UseKiTs=off  D=0.01  N=100  UseFilter=on  TunerSelectOption=Transfer Function Based (PID Tuner App)  InitialConditionSource=internal  InitialConditionForIntegrator=0  InitialConditionForFilter=0  DifferentiatorICPrevScaledInput=0  ExternalReset=either  TrackingMode=off  Kt=1  LimitOutput=off  SatLimitsSource=internal  UpperSaturationLimit=inf  LowerSaturationLimit=-inf  LinearizeAsGain=on  AntiWindupMode=none  Kb=1  LimitIntegrator=off  UpperIntegratorSaturationLimit=inf  LowerIntegratorSaturationLimit=-inf  POutMin=[]  POutMax=[]  IOutMin=[]  IOutMax=[]  DOutMin=[]  DOutMax=[]  NOutMin=[]  NOutMax=[]  SumOutMin=[]  SumOutMax=[]  SaturationOutMin=[]  SaturationOutMax=[]  PParamMin=[]  PParamMax=[]  IParamMin=[]  IParamMax=[]  DParamMin=[]  DParamMax=[]  NParamMin=[]  NParamMax=[]  KbParamMin=[]  KbParamMax=[]  KtParamMin=[]  KtParamMax=[]  KbOutMin=[]  KbOutMax=[]  KtOutMin=[]  KtOutMax=[]  IntegratorOutMin=[]  IntegratorOutMax=[]  FilterOutMin=[]  FilterOutMax=[]  SumI1OutMin=[]  SumI1OutMax=[]  SumI2OutMin=[]  SumI2OutMax=[]  SumI3OutMin=[]  SumI3OutMax=[]  SumI4OutMin=[]  SumI4OutMax=[]  SumDOutMin=[]  SumDOutMax=[]  DifferentiatorOutMin=[]  DifferentiatorOutMax=[]  FilterDiffOutCoefMin=[]  FilterDiffOutCoefMax=[]  ReciprocalOutMin=[]  ReciprocalOutMax=[]  SumDenOutMin=[]  SumDenOutMax=[]  SumNumOutMin=[]  SumNumOutMax=[]  DivideOutMin=[]  DivideOutMax=[]  UdiffTsProdOutMin=[]  UdiffTsProdOutMax=[]  NTsProdOutMin=[]  NTsProdOutMax=[]  UintegralTsProdOutMin=[]  UintegralTsProdOutMax=[]  UngainTsProdOutMin=[]  UngainTsProdOutMax=[]  ClampingZeroOutDataTypeStr=Inherit: Inherit via back propagation  ClampingZeroOutMin=[]  ClampingZeroOutMax=[]  FilterDenConstantOutDataTypeStr=Inherit: Inherit via back propagation  FilterDenConstantOutMin=[]  FilterDenConstantOutMax=[]  PCopyOutDataTypeStr=Inherit: Inherit via back propagation  PCopyOutMin=[]  PCopyOutMax=[]  NCopyOutDataTypeStr=Inherit: Inherit via back propagation  NCopyOutMin=[]  NCopyOutMax=[]  IntegratorContinuousStateAttributes=''  IntegratorStateMustResolveToSignalObject=off  IntegratorRTWStateStorageClass=Auto  FilterContinuousStateAttributes=''  FilterStateMustResolveToSignalObject=off  FilterRTWStateStorageClass=Auto  ParallelPVariant=InternalParameters  IdealPVariant=Disabled  IVariant=InternalParameters  DVariant=Disabled  IntegratorVariant=Continuous  SatVariant=Disabled  AWVariant=Passthrough  PCopyVariant=Disabled  TRVariant=Disabled  FdbkBlocksVariant=Forward  IdealPFdbkVariant=Disabled  SatFdbkVariant=Disabled  DerivativeFilterVariant=Disabled  NVariant=Disabled  NCopyVariant=Disabled_SignalSpec  FilterICVariant=Disabled  IntegratorICVariant=InternalICs  ExternalResetVariant=ExternalReset  TRSumVariant=Passthrough  SumFdbkVariant=Disabled  SumVariant=Sum_PI  TsampFilterVariant=InternalTs  TsampNgainVariant=Passthrough  TsampIntegralVariant=Disabled_SignalSpec  ExternalSaturationOutDataTypeStr=Inherit: Same as second input
  Subsystem1 : $bdroot/SVR Control/Subsystem1  SystemSampleTime=-1  VariantActivationTime=update diagram  Latency=0  AutoFrameSizeCalculation=off
  Subsystem2 : $bdroot/SVR Control/Subsystem2  SystemSampleTime=-1  VariantActivationTime=update diagram  Latency=0  AutoFrameSizeCalculation=off
  Subtract : Sum  Inputs=-+
  Switch : Switch  Criteria=u2 > Threshold  SaturateOnIntegerOverflow=off  InputSameDT=off
  Switch1 : Switch  Criteria=u2 > Threshold  SaturateOnIntegerOverflow=off  InputSameDT=off
  Switch2 : Switch  Criteria=u2 > Threshold  SaturateOnIntegerOverflow=off  InputSameDT=off
  Unit Delay2 : UnitDelay  SampleTime=-1  HasFrameUpgradeWarning=on
  wires:
  Switch/1 -> Subtract/2
  Subtract/1 -> PID Controller/1  "V(t)"
  [PVR] -> Subsystem1/1, Switch/3
  Switch1/1 -> Subtract/1, Switch/1
  Subsystem1/1 -> Switch/2
  Constant/1 -> Switch1/3
  Constant1/1 -> OR/1
  PVR(t)/1 -> Switch1/2, IsZero1/1, Switch1/1
  IsZero1/1 -> OR/2
  Switch2/1 -> Data Store Write/1
  K_pvr/1 -> Switch2/3
  OR/1 -> PID Controller/2, MATLAB Function/Trigger, Unit Delay2/1, Subsystem2/2
  PID Controller/1 -> Subsystem2/1
  Unit Delay2/1 -> Switch2/2
  Subsystem2/1 -> MATLAB Function/1(u), Switch2/1

== system Vessel/Radius ==
  V(t) : Inport  Unit=mL
  Gain : Gain  Gain=1/(pi*l*n)
  Gain1 : $bdroot/Gain  SystemSampleTime=-1  VariantActivationTime=update diagram  Latency=0  AutoFrameSizeCalculation=off
  Product : Product
  Sqrt : Sqrt
  r(t) : Outport  Unit=cm
  wires:
  Gain/1 -> Sqrt/1
  Sqrt/1 -> Product/1
  V(t)/1 -> Gain/1
  Gain1/1 -> Product/2
  Product/1 -> r(t)/1

== system Vessel/Resistance ==
  r(t) : Inport
  Gain : Gain  Gain=eta*8*l/(pi*n)*1.1732
  Math Function : Math  Operator=reciprocal
  Power : Math  Operator=square
  Power1 : Math  Operator=square
  R(t) : Outport
  wires:
  r(t)/1 -> Power/1
  Power/1 -> Power1/1
  Power1/1 -> Math Function/1
  Math Function/1 -> Gain/1
  Gain/1 -> R(t)/1  "R(t)"

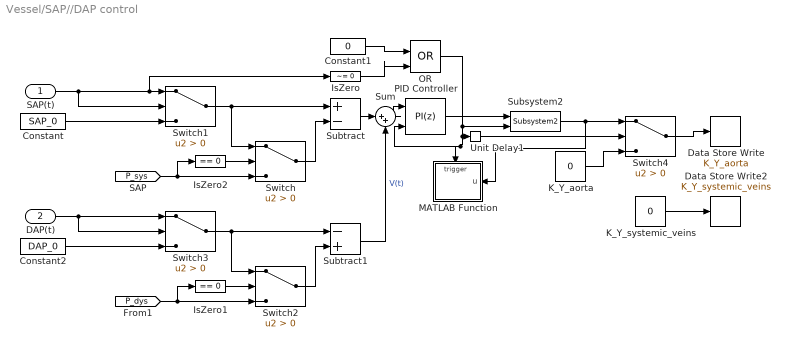
== system Vessel/SAP//DAP control ==
  SAP(t) : Inport
  DAP(t) : Inport  Port=2
  Constant : Constant  Value=SAP_0
  Constant1 : Constant  Value=0
  Constant2 : Constant  Value=DAP_0
  Data Store Write : DataStoreWrite  DataStoreName=K_Y_aorta  IndexOptions=Index vector (dialog)  Indices=1  OutputSizes=1
  Data Store Write2 : DataStoreWrite  DataStoreName=K_Y_systemic_veins  IndexOptions=Index vector (dialog)  Indices=1  OutputSizes=1
  IsZero : simulink/Logic and Bit Operations/Compare To Zero  relop=~=  OutDataTypeStr=boolean
      settings: LibrarySourceBlock=|
      | simulink/Quick Insert/Logic and Bit
      | Operations/IsZero
  IsZero1 : simulink/Logic and Bit Operations/Compare To Zero  relop===  OutDataTypeStr=boolean
      settings: LibrarySourceBlock=|
      | simulink/Quick Insert/Logic and Bit
      | Operations/IsZero
  IsZero2 : simulink/Logic and Bit Operations/Compare To Zero  relop===  OutDataTypeStr=boolean
      settings: LibrarySourceBlock=|
      | simulink/Quick Insert/Logic and Bit
      | Operations/IsZero
  K_Y_aorta : Constant  Value=0
  K_Y_systemic_veins : Constant  Value=0
  MATLAB Function : MATLAB Function  TreatAsAtomicUnit=on
  OR : Logic  Operator=OR  IconShape=distinctive  AllPortsSameDT=off  OutDataTypeStr=boolean
  PID Controller : slpidlib/PID Controller  Controller=PI  Form=Parallel  TimeDomain=Discrete-time  UseExternalTs=off  SampleTime=dt  IntegratorMethod=Forward Euler  FilterMethod=Forward Euler  ControllerParametersSource=internal  P=0.01  I=0.01  UseKiTs=off  D=0.01  N=100  UseFilter=on  TunerSelectOption=Transfer Function Based (PID Tuner App)  InitialConditionSource=internal  InitialConditionForIntegrator=0  InitialConditionForFilter=0  DifferentiatorICPrevScaledInput=0  ExternalReset=either  TrackingMode=off  Kt=1  LimitOutput=on  SatLimitsSource=internal  UpperSaturationLimit=2  LowerSaturationLimit=-0.99  LinearizeAsGain=on  AntiWindupMode=none  Kb=1  LimitIntegrator=off  UpperIntegratorSaturationLimit=inf  LowerIntegratorSaturationLimit=-inf  POutMin=[]  POutMax=[]  IOutMin=[]  IOutMax=[]  DOutMin=[]  DOutMax=[]  NOutMin=[]  NOutMax=[]  SumOutMin=[]  SumOutMax=[]  SaturationOutMin=[]  SaturationOutMax=[]  PParamMin=[]  PParamMax=[]  IParamMin=[]  IParamMax=[]  DParamMin=[]  DParamMax=[]  NParamMin=[]  NParamMax=[]  KbParamMin=[]  KbParamMax=[]  KtParamMin=[]  KtParamMax=[]  KbOutMin=[]  KbOutMax=[]  KtOutMin=[]  KtOutMax=[]  IntegratorOutMin=[]  IntegratorOutMax=[]  FilterOutMin=[]  FilterOutMax=[]  SumI1OutMin=[]  SumI1OutMax=[]  SumI2OutMin=[]  SumI2OutMax=[]  SumI3OutMin=[]  SumI3OutMax=[]  SumI4OutMin=[]  SumI4OutMax=[]  SumDOutMin=[]  SumDOutMax=[]  DifferentiatorOutMin=[]  DifferentiatorOutMax=[]  FilterDiffOutCoefMin=[]  FilterDiffOutCoefMax=[]  ReciprocalOutMin=[]  ReciprocalOutMax=[]  SumDenOutMin=[]  SumDenOutMax=[]  SumNumOutMin=[]  SumNumOutMax=[]  DivideOutMin=[]  DivideOutMax=[]  UdiffTsProdOutMin=[]  UdiffTsProdOutMax=[]  NTsProdOutMin=[]  NTsProdOutMax=[]  UintegralTsProdOutMin=[]  UintegralTsProdOutMax=[]  UngainTsProdOutMin=[]  UngainTsProdOutMax=[]  ClampingZeroOutDataTypeStr=Inherit: Inherit via back propagation  ClampingZeroOutMin=[]  ClampingZeroOutMax=[]  FilterDenConstantOutDataTypeStr=Inherit: Inherit via back propagation  FilterDenConstantOutMin=[]  FilterDenConstantOutMax=[]  PCopyOutDataTypeStr=Inherit: Inherit via back propagation  PCopyOutMin=[]  PCopyOutMax=[]  NCopyOutDataTypeStr=Inherit: Inherit via back propagation  NCopyOutMin=[]  NCopyOutMax=[]  IntegratorContinuousStateAttributes=''  IntegratorStateMustResolveToSignalObject=off  IntegratorRTWStateStorageClass=Auto  FilterContinuousStateAttributes=''  FilterStateMustResolveToSignalObject=off  FilterRTWStateStorageClass=Auto  ParallelPVariant=InternalParameters  IdealPVariant=Disabled  IVariant=InternalParameters  DVariant=Disabled  IntegratorVariant=Discrete  SatVariant=Enabled  AWVariant=Passthrough  PCopyVariant=Disabled  TRVariant=Disabled  FdbkBlocksVariant=Forward  IdealPFdbkVariant=Disabled  SatFdbkVariant=Disabled  DerivativeFilterVariant=Disabled  NVariant=Disabled  NCopyVariant=Disabled_SignalSpec  FilterICVariant=Disabled  IntegratorICVariant=InternalICs  ExternalResetVariant=ExternalReset  TRSumVariant=Passthrough  SumFdbkVariant=Disabled  SumVariant=Sum_PI  TsampFilterVariant=InternalTs  TsampNgainVariant=Passthrough  TsampIntegralVariant=Disabled_SignalSpec  ExternalSaturationOutDataTypeStr=Inherit: Same as second input
  Subsystem2 : $bdroot/SVR Control/Subsystem2  SystemSampleTime=-1  VariantActivationTime=update diagram  Latency=0  AutoFrameSizeCalculation=off
  Subtract : Sum  Inputs=+-
  Subtract1 : Sum  Inputs=-+
  Sum : Sum  Inputs=|++
  Switch{,1..4} (5 alike) : Switch  Criteria=u2 > Threshold  SaturateOnIntegerOverflow=off  InputSameDT=off
  Unit Delay1 : UnitDelay  SampleTime=-1  HasFrameUpgradeWarning=on
  wires:
  Constant/1 -> Switch1/3
  [P_sys] -> IsZero2/1, Switch/3
  Switch/1 -> Subtract/2
  IsZero2/1 -> Switch/2
  SAP(t)/1 -> Switch1/2, IsZero/1, Switch1/1
  Switch1/1 -> Subtract/1, Switch/1
  IsZero/1 -> OR/2
  Constant1/1 -> OR/1
  [P_dys] -> IsZero1/1, Switch2/3
  DAP(t)/1 -> Switch3/1, Switch3/2
  Switch2/1 -> Subtract1/2
  IsZero1/1 -> Switch2/2
  Subtract1/1 -> Sum/2  "V(t)"
  Constant2/1 -> Switch3/3
  Switch3/1 -> Switch2/1, Subtract1/1
  Subtract/1 -> Sum/1
  Sum/1 -> PID Controller/1
  Switch4/1 -> Data Store Write/1
  K_Y_aorta/1 -> Switch4/3
  K_Y_systemic_veins/1 -> Data Store Write2/1
  OR/1 -> Unit Delay1/1, PID Controller/2, MATLAB Function/Trigger, Subsystem2/2
  PID Controller/1 -> Subsystem2/1
  Subsystem2/1 -> Switch4/1, MATLAB Function/1(u)
  Unit Delay1/1 -> Switch4/2

== system Vessel/SLVP control ==
  SLVP(t) : Inport
  Constant : Constant  Value=SLVP_0
  Constant1 : Constant  Value=0
  Data Store Write : DataStoreWrite  DataStoreName=K_LV_Emax  IndexOptions=Index vector (dialog)  Indices=1  OutputSizes=1
  Data Store Write11 : DataStoreWrite  DataStoreName=K_LV_Emin  IndexOptions=Index vector (dialog)  Indices=1  OutputSizes=1
  Data Store Write7 : DataStoreWrite  DataStoreName=K_LA_Emax  IndexOptions=Index vector (dialog)  Indices=1  OutputSizes=1
  Data Store Write8 : DataStoreWrite  DataStoreName=K_LA_Emin  IndexOptions=Index vector (dialog)  Indices=1  OutputSizes=1
  IsZero : simulink/Logic and Bit Operations/Compare To Zero  relop=~=  OutDataTypeStr=boolean
      settings: LibrarySourceBlock=|
      | simulink/Quick Insert/Logic and Bit
      | Operations/IsZero
  IsZero2 : simulink/Logic and Bit Operations/Compare To Zero  relop===  OutDataTypeStr=boolean
      settings: LibrarySourceBlock=|
      | simulink/Quick Insert/Logic and Bit
      | Operations/IsZero
  K_LA_Emax : Constant  Value=0
  K_LA_Emin : Constant  Value=0
  K_LV_Emax : Constant  Value=0
  K_LV_Emin : Constant  Value=0
  MATLAB Function : MATLAB Function  TreatAsAtomicUnit=on
  OR : Logic  Operator=OR  IconShape=distinctive  AllPortsSameDT=off  OutDataTypeStr=boolean
  PID Controller : slpidlib/PID Controller  Controller=PI  Form=Parallel  TimeDomain=Discrete-time  UseExternalTs=off  SampleTime=dt  IntegratorMethod=Forward Euler  FilterMethod=Forward Euler  ControllerParametersSource=internal  P=0.005  I=0.005  UseKiTs=off  D=0.01  N=100  UseFilter=on  TunerSelectOption=Transfer Function Based (PID Tuner App)  InitialConditionSource=internal  InitialConditionForIntegrator=0  InitialConditionForFilter=0  DifferentiatorICPrevScaledInput=0  ExternalReset=either  TrackingMode=off  Kt=1  LimitOutput=on  SatLimitsSource=internal  UpperSaturationLimit=2  LowerSaturationLimit=-0.99  LinearizeAsGain=on  AntiWindupMode=none  Kb=1  LimitIntegrator=off  UpperIntegratorSaturationLimit=inf  LowerIntegratorSaturationLimit=-inf  POutMin=[]  POutMax=[]  IOutMin=[]  IOutMax=[]  DOutMin=[]  DOutMax=[]  NOutMin=[]  NOutMax=[]  SumOutMin=[]  SumOutMax=[]  SaturationOutMin=[]  SaturationOutMax=[]  PParamMin=[]  PParamMax=[]  IParamMin=[]  IParamMax=[]  DParamMin=[]  DParamMax=[]  NParamMin=[]  NParamMax=[]  KbParamMin=[]  KbParamMax=[]  KtParamMin=[]  KtParamMax=[]  KbOutMin=[]  KbOutMax=[]  KtOutMin=[]  KtOutMax=[]  IntegratorOutMin=[]  IntegratorOutMax=[]  FilterOutMin=[]  FilterOutMax=[]  SumI1OutMin=[]  SumI1OutMax=[]  SumI2OutMin=[]  SumI2OutMax=[]  SumI3OutMin=[]  SumI3OutMax=[]  SumI4OutMin=[]  SumI4OutMax=[]  SumDOutMin=[]  SumDOutMax=[]  DifferentiatorOutMin=[]  DifferentiatorOutMax=[]  FilterDiffOutCoefMin=[]  FilterDiffOutCoefMax=[]  ReciprocalOutMin=[]  ReciprocalOutMax=[]  SumDenOutMin=[]  SumDenOutMax=[]  SumNumOutMin=[]  SumNumOutMax=[]  DivideOutMin=[]  DivideOutMax=[]  UdiffTsProdOutMin=[]  UdiffTsProdOutMax=[]  NTsProdOutMin=[]  NTsProdOutMax=[]  UintegralTsProdOutMin=[]  UintegralTsProdOutMax=[]  UngainTsProdOutMin=[]  UngainTsProdOutMax=[]  ClampingZeroOutDataTypeStr=Inherit: Inherit via back propagation  ClampingZeroOutMin=[]  ClampingZeroOutMax=[]  FilterDenConstantOutDataTypeStr=Inherit: Inherit via back propagation  FilterDenConstantOutMin=[]  FilterDenConstantOutMax=[]  PCopyOutDataTypeStr=Inherit: Inherit via back propagation  PCopyOutMin=[]  PCopyOutMax=[]  NCopyOutDataTypeStr=Inherit: Inherit via back propagation  NCopyOutMin=[]  NCopyOutMax=[]  IntegratorContinuousStateAttributes=''  IntegratorStateMustResolveToSignalObject=off  IntegratorRTWStateStorageClass=Auto  FilterContinuousStateAttributes=''  FilterStateMustResolveToSignalObject=off  FilterRTWStateStorageClass=Auto  ParallelPVariant=InternalParameters  IdealPVariant=Disabled  IVariant=InternalParameters  DVariant=Disabled  IntegratorVariant=Discrete  SatVariant=Enabled  AWVariant=Passthrough  PCopyVariant=Disabled  TRVariant=Disabled  FdbkBlocksVariant=Forward  IdealPFdbkVariant=Disabled  SatFdbkVariant=Disabled  DerivativeFilterVariant=Disabled  NVariant=Disabled  NCopyVariant=Disabled_SignalSpec  FilterICVariant=Disabled  IntegratorICVariant=InternalICs  ExternalResetVariant=ExternalReset  TRSumVariant=Passthrough  SumFdbkVariant=Disabled  SumVariant=Sum_PI  TsampFilterVariant=InternalTs  TsampNgainVariant=Passthrough  TsampIntegralVariant=Disabled_SignalSpec  ExternalSaturationOutDataTypeStr=Inherit: Same as second input
  Subsystem2 : $bdroot/SVR Control/Subsystem2  SystemSampleTime=-1  VariantActivationTime=update diagram  Latency=0  AutoFrameSizeCalculation=off
  Subtract : Sum  Inputs=+-
  Switch : Switch  Criteria=u2 > Threshold  SaturateOnIntegerOverflow=off  InputSameDT=off
  Switch1 : Switch  Criteria=u2 > Threshold  SaturateOnIntegerOverflow=off  InputSameDT=off
  Switch2 : Switch  Criteria=u2 > Threshold  SaturateOnIntegerOverflow=off  InputSameDT=off
  Unit Delay2 : UnitDelay  SampleTime=-1  HasFrameUpgradeWarning=on
  wires:
  Constant1/1 -> OR/1
  IsZero/1 -> OR/2
  Switch1/1 -> Switch/1, Subtract/1
  SLVP(t)/1 -> Switch1/1, IsZero/1, Switch1/2
  IsZero2/1 -> Switch/2
  Switch/1 -> Subtract/2
  [MAP] -> IsZero2/1, Switch/3
  Constant/1 -> Switch1/3
  Subtract/1 -> PID Controller/1  "V(t)"
  Switch2/1 -> Data Store Write/1
  K_LV_Emin/1 -> Data Store Write11/1
  K_LV_Emax/1 -> Switch2/3
  K_LA_Emin/1 -> Data Store Write8/1
  K_LA_Emax/1 -> Data Store Write7/1
  OR/1 -> Unit Delay2/1, PID Controller/2, MATLAB Function/Trigger, Subsystem2/2
  PID Controller/1 -> Subsystem2/1
  Unit Delay2/1 -> Switch2/2
  Subsystem2/1 -> MATLAB Function/1(u), Switch2/1
